simulink library "Storage_Type_1_CONF"  (Simulink 8.2)
settings: Solver=ode45  StartTime=0.0  StopTime=10.0  RelTol=1e-3
libraries: carnot x2
settings Model: Creator=lena.frank  LastModifiedBy=drhf

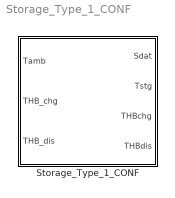
== system Storage_Type_1_CONF ==
  Storage_Type_1_CONF : Subsystem  mask(Buffer Storage with 2 connections){parameterfile=default_Storage, tini=[10:5:55]}
      mask prompts: parameterfile "Storage parameter set"; tini "initial temperature (vector or scalar) in °C"
      mask help: Predefinded storage with 2 direct ports (for example a buffer storage tank).
      mask init:
      | % callback to set parameters of model
      | CarnotCallbacks_StorageConf(1,parameterfile);
      mask Help: web(fullfile(path_carnot('help'),'Storage_Type_N.html'),'-helpbrowser')
      mask TypeOptions parameterfile: default_Storage
      mask Display:
      | % user defined picture file
      | picfile = fullfile(path_carnot('intlibsl'), ...
      |     'Storage','Thermal','Storage_Type_1_CONF','parameter_set', ...
      |     'Storage_Type_1_CONF.jpg');
      | 
      | % show public picture
      | plot([40,40,45,55,60,60,55,45,40]/100,[84,36,30,30,36,84,90,90,84]/100, ...
      |     [40,35]/100,[77,77]/100,[64,60]/100,[77,77]/100,[40,35]/100,[42,42]/100, ...
      |     [64,60]/100,[42,42]/100)
      | 
      | % show internal picture if defined
      | if ~BlockIsInCarnotLibrary    % if not located in library any more
      |     if exist(picfile)
      |         image(imread(picfile), [0.3, 0, 0.5, 1])
      |         set_param(gcb, 'BackgroundColor', 'White')
      |     end
      | end

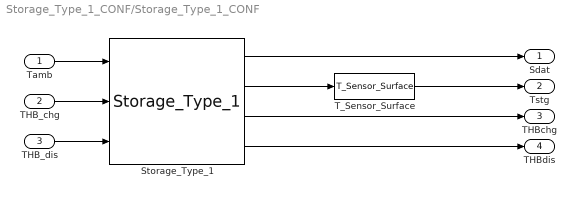
== system Storage_Type_1_CONF/Storage_Type_1_CONF ==
  Tamb : Inport
  THB_chg : Inport  Port=2
  THB_dis : Inport  Port=3
  Storage_Type_1 : carnot/Storage/Thermal/Storage_Type_1  uloss=1  ubot=1  utop=1  cond=1  t0=tini  volume=0.3  dia=0.5  pos=standing cylinder  nconnect=2  nodes=10  mpoints=10
  T_Sensor_Surface : carnot/Control/T_Sensor_Surface  pos=[0.5]  tdel=10  t0=tini(1)
  Sdat : Outport
  Tstg : Outport  Port=2
  THBchg : Outport  Port=3
  THBdis : Outport  Port=4
  wires:
  Storage_Type_1/4 -> THBdis/1
  Storage_Type_1/3 -> THBchg/1
  Storage_Type_1/2 -> T_Sensor_Surface/1
  Storage_Type_1/1 -> Sdat/1
  THB_dis/1 -> Storage_Type_1/3
  THB_chg/1 -> Storage_Type_1/2
  Tamb/1 -> Storage_Type_1/1
  T_Sensor_Surface/1 -> Tstg/1
